simulink model "switching_mask"  (R2018a)
settings: Solver=FixedStepAuto  StartTime=0.0  StopTime=0.08  FixedStep=2.5000e-06  RelTol=1e-3
libraries: powerlib_meascontrol x11
settings Model: Creator=enes_  LastModifiedBy=enes_

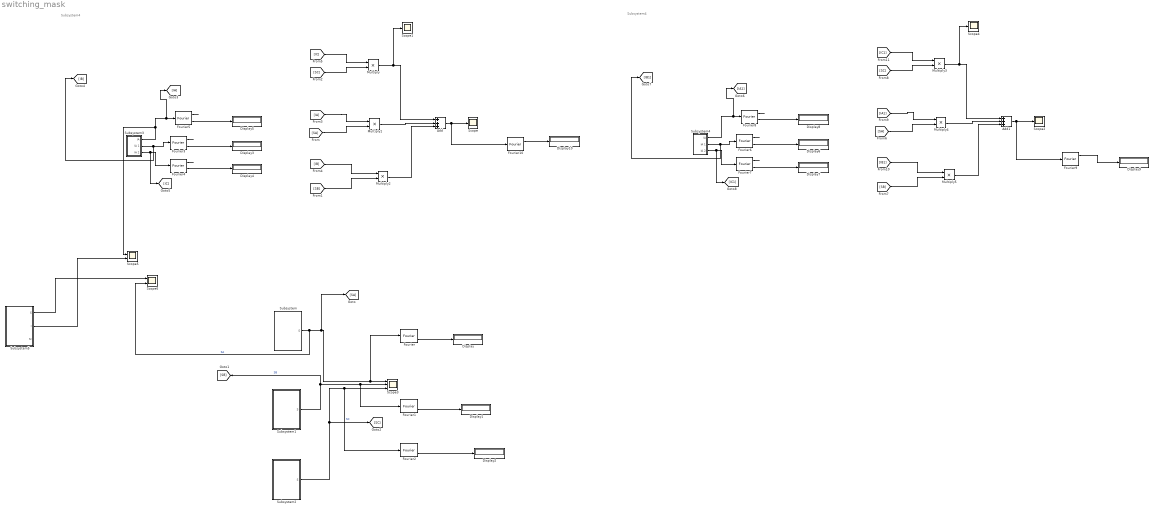
== system switching_mask ==
  note: Subsystem4
  note: Subsystem4
  Add : Sum  Inputs=3
  Add1 : Sum  Inputs=3
  Display{,1..10} (11 alike) : Display
  Fourier{,1..8} (9 alike) : powerlib_meascontrol/Measurements/Fourier  Freq=50  n=1  InInit=[0, 0]  Ts=0
      settings: SourceProductName=Simscape Power Systems
  Fourier10 : powerlib_meascontrol/Measurements/Fourier  Freq=100  n=1  InInit=[0, 0]  Ts=0
      settings: SourceProductName=Simscape Power Systems
  Fourier9 : powerlib_meascontrol/Measurements/Fourier  Freq=100  n=1  InInit=[0, 0]  Ts=0
      settings: SourceProductName=Simscape Power Systems
  Multiply{,1..5} (6 alike) : Product
  Scope{,1..2,4} (4 alike) : Scope
  Scope3 : Scope  NumInputPorts=3
  Scope5 : Scope  NumInputPorts=2
  Scope6 : Scope  NumInputPorts=2
  Subsystem : Subsystem  mask{m=0.9, f_s=4e4, f_f=50, the_f=0, the_c=0, i1=20, i2=5}
      mask prompts: m "modulation index"; f_s "carrier frequency"; f_f "fundemental frequency"; the_f "phase of fundamental"; the_c "phase of carrier"; i1 "iteration number of carrier"; i2 "iteration number of fundamental"
  Subsystem1 : Subsystem  mask{m=0.9, f_s=4e4, f_f=50, the_f=2*pi/3, the_c=0, i1=20, i2=5}
      mask prompts: m "modulation index"; f_s "carrier frequency"; f_f "fundemental frequency"; the_f "phase of fundamental"; the_c "phase of carrier"; i1 "iteration number of carrier"; i2 "iteration number of fundamental"
  Subsystem2 : Subsystem  mask{m=0.9, f_s=4e4, f_f=50, the_f=4*pi/3, the_c=0, i1=20, i2=5}
      mask prompts: m "modulation index"; f_s "carrier frequency"; f_f "fundemental frequency"; the_f "phase of fundamental"; the_c "phase of carrier"; i1 "iteration number of carrier"; i2 "iteration number of fundamental"
  Subsystem3 : Subsystem
  Subsystem4 : Subsystem
  Subsystem5 : Subsystem  mask{m=0.9, f_s=4e4, f_f=50, the_f=0, the_c=0, i1=20, i2=5, load_phase=pi/6}
      mask prompts: m "modulation index"; f_s "carrier frequency"; f_f "fundemental frequency"; the_f "phase of fundamental"; the_c "phase of carrier"; i1 "iteration number of carrier"; i2 "iteration number of fundamental"; load_phase "phase of load current"
  wires:
  Subsystem/1(S) -> Scope6/2, [SA], Fourier/1, Scope3/1  "SA"
  Subsystem1/1(S) -> [SB], Fourier1/1, Scope3/2  "SB"
  Subsystem2/1(S) -> [SC], Fourier2/1, Scope3/3  "SC"
  Fourier/2 -> Display/1
  Fourier1/2 -> Display1/1
  Fourier2/2 -> Display2/1
  Fourier3/1 -> ?
  [SC] -> Multiply/2
  [IA] -> Multiply1/1
  Subsystem3/1("IA ") -> Scope5/1, [IA], Fourier5/1
  Fourier5/2 -> Display5/1
  Multiply/1 -> Scope1/1, Add/1
  Fourier4/2 -> Display4/1
  Multiply1/1 -> Add/2
  [SB] -> Multiply2/2
  Fourier4/1 -> ?
  [SA] -> Multiply1/2
  [IB] -> Multiply2/1
  Subsystem3/2(IA 1) -> [IB], Fourier3/1
  Fourier5/1 -> ?
  Subsystem3/3(IA 2) -> [IC], Fourier4/1
  Multiply2/1 -> Add/3
  [IC] -> Multiply/1
  Fourier3/2 -> Display3/1
  Multiply3/1 -> Scope4/1, Add1/1
  [SC] -> Multiply3/2
  [IB1] -> Multiply5/1
  Fourier7/2 -> Display7/1
  Subsystem4/1("IA ") -> [IA1], Fourier8/1
  [IA1] -> Multiply4/1
  Fourier8/2 -> Display8/1
  Subsystem4/2(IA 1) -> [IB1], Fourier6/1
  Multiply5/1 -> Add1/3
  Subsystem4/3(IA 2) -> [IC1], Fourier7/1
  [SA] -> Multiply4/2
  Multiply4/1 -> Add1/2
  Fourier8/1 -> ?
  [SB] -> Multiply5/2
  Fourier6/1 -> ?
  Fourier6/2 -> Display6/1
  [IC1] -> Multiply3/1
  Fourier7/1 -> ?
  Add1/1 -> Fourier9/1, Scope2/1
  Fourier9/1 -> Display9/1
  Fourier10/1 -> Display10/1
  Add/1 -> Fourier10/1, Scope/1
  Subsystem5/2("I ") -> Scope5/2
  Subsystem5/1(S) -> Scope6/1

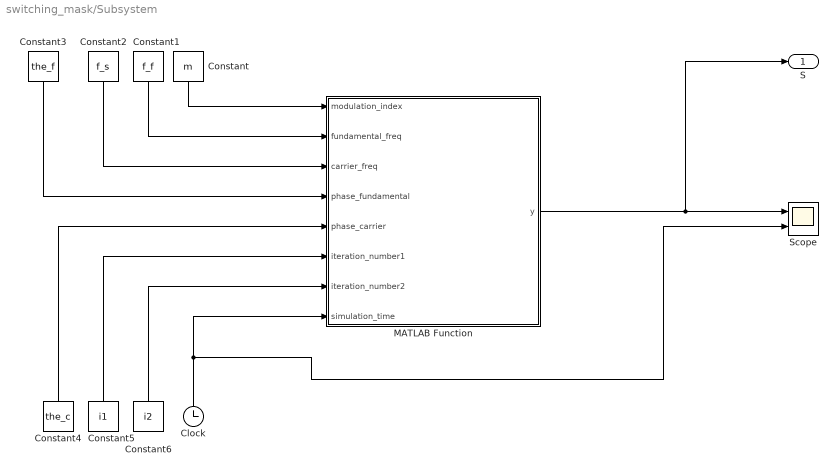
== system switching_mask/Subsystem ==
  Clock : Clock
  Constant : Constant  Value=m
  Constant1 : Constant  Value=f_f
  Constant2 : Constant  Value=f_s
  Constant3 : Constant  Value=the_f
  Constant4 : Constant  Value=the_c
  Constant5 : Constant  Value=i1
  Constant6 : Constant  Value=i2
  MATLAB Function : MATLAB Function  TreatAsAtomicUnit=on
  Scope : Scope  NumInputPorts=2
  S : Outport
  wires:
  Constant/1 -> MATLAB Function/1(modulation_index)
  Constant1/1 -> MATLAB Function/2(fundamental_freq)
  Constant2/1 -> MATLAB Function/3(carrier_freq)
  Constant3/1 -> MATLAB Function/4(phase_fundamental)
  Constant4/1 -> MATLAB Function/5(phase_carrier)
  Constant5/1 -> MATLAB Function/6(iteration_number1)
  Constant6/1 -> MATLAB Function/7(iteration_number2)
  MATLAB Function/1(y) -> S/1, Scope/1
  Clock/1 -> Scope/2, MATLAB Function/8(simulation_time)

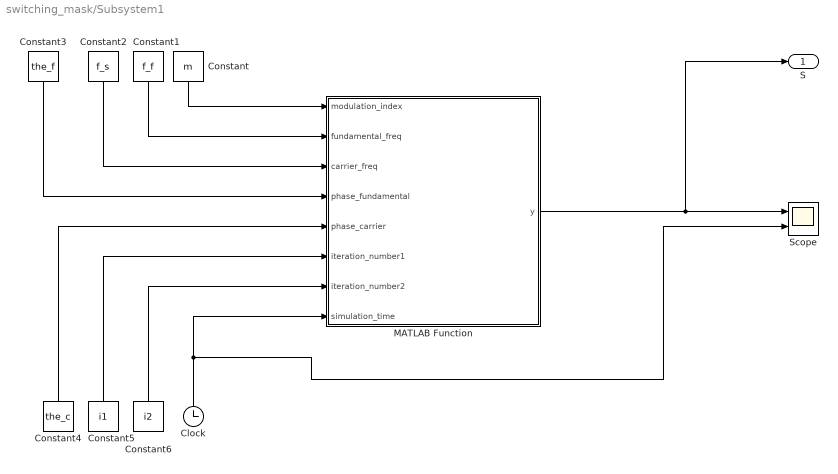
== system switching_mask/Subsystem1 ==
  Clock : Clock
  Constant : Constant  Value=m
  Constant1 : Constant  Value=f_f
  Constant2 : Constant  Value=f_s
  Constant3 : Constant  Value=the_f
  Constant4 : Constant  Value=the_c
  Constant5 : Constant  Value=i1
  Constant6 : Constant  Value=i2
  MATLAB Function : MATLAB Function  TreatAsAtomicUnit=on
  Scope : Scope  NumInputPorts=2
  S : Outport
  wires:
  Constant/1 -> MATLAB Function/1(modulation_index)
  Constant1/1 -> MATLAB Function/2(fundamental_freq)
  Constant2/1 -> MATLAB Function/3(carrier_freq)
  Constant3/1 -> MATLAB Function/4(phase_fundamental)
  Constant4/1 -> MATLAB Function/5(phase_carrier)
  Constant5/1 -> MATLAB Function/6(iteration_number1)
  Constant6/1 -> MATLAB Function/7(iteration_number2)
  MATLAB Function/1(y) -> S/1, Scope/1
  Clock/1 -> Scope/2, MATLAB Function/8(simulation_time)

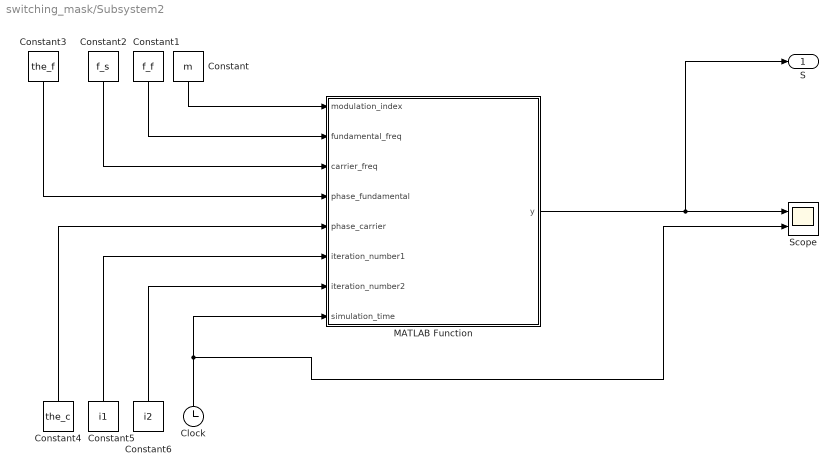
== system switching_mask/Subsystem2 ==
  Clock : Clock
  Constant : Constant  Value=m
  Constant1 : Constant  Value=f_f
  Constant2 : Constant  Value=f_s
  Constant3 : Constant  Value=the_f
  Constant4 : Constant  Value=the_c
  Constant5 : Constant  Value=i1
  Constant6 : Constant  Value=i2
  MATLAB Function : MATLAB Function  TreatAsAtomicUnit=on
  Scope : Scope  NumInputPorts=2
  S : Outport
  wires:
  Constant/1 -> MATLAB Function/1(modulation_index)
  Constant1/1 -> MATLAB Function/2(fundamental_freq)
  Constant2/1 -> MATLAB Function/3(carrier_freq)
  Constant3/1 -> MATLAB Function/4(phase_fundamental)
  Constant4/1 -> MATLAB Function/5(phase_carrier)
  Constant5/1 -> MATLAB Function/6(iteration_number1)
  Constant6/1 -> MATLAB Function/7(iteration_number2)
  MATLAB Function/1(y) -> S/1, Scope/1
  Clock/1 -> Scope/2, MATLAB Function/8(simulation_time)

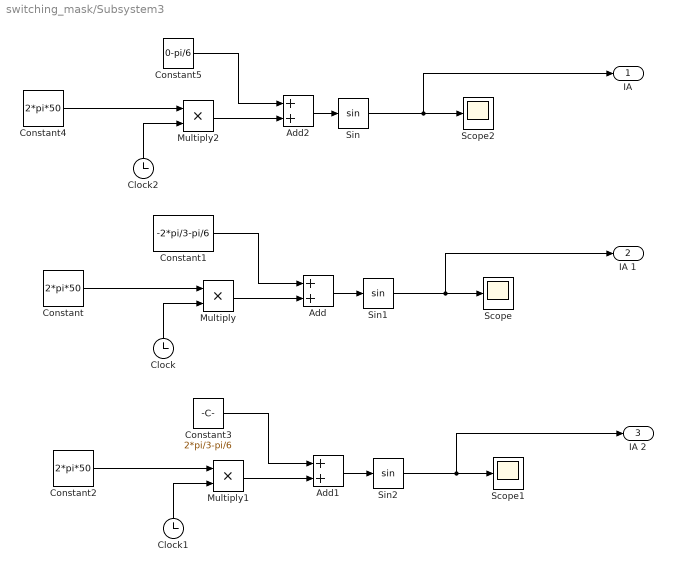
== system switching_mask/Subsystem3 ==
  Add : Sum
  Add1 : Sum
  Add2 : Sum
  Clock : Clock
  Clock1 : Clock
  Clock2 : Clock
  Constant : Constant  Value=2*pi*50
  Constant1 : Constant  Value=-2*pi/3-pi/6
  Constant2 : Constant  Value=2*pi*50
  Constant3 : Constant  Value=2*pi/3-pi/6
  Constant4 : Constant  Value=2*pi*50
  Constant5 : Constant  Value=0-pi/6
  Multiply : Product
  Multiply1 : Product
  Multiply2 : Product
  Scope : Scope
  Scope1 : Scope
  Scope2 : Scope
  Sin : Trigonometry
  Sin1 : Trigonometry
  Sin2 : Trigonometry
  "IA " : Outport
  IA 1 : Outport  Port=2
  IA 2 : Outport  Port=3
  wires:
  Multiply2/1 -> Add2/2
  Sin2/1 -> IA 2/1, Scope1/1
  Clock/1 -> Multiply/2
  Sin1/1 -> IA 1/1, Scope/1
  Sin/1 -> "IA "/1, Scope2/1
  Constant4/1 -> Multiply2/1
  Add/1 -> Sin1/1
  Constant3/1 -> Add1/1
  Clock2/1 -> Multiply2/2
  Add1/1 -> Sin2/1
  Constant2/1 -> Multiply1/1
  Clock1/1 -> Multiply1/2
  Multiply1/1 -> Add1/2
  Add2/1 -> Sin/1
  Constant1/1 -> Add/1
  Constant5/1 -> Add2/1
  Multiply/1 -> Add/2
  Constant/1 -> Multiply/1

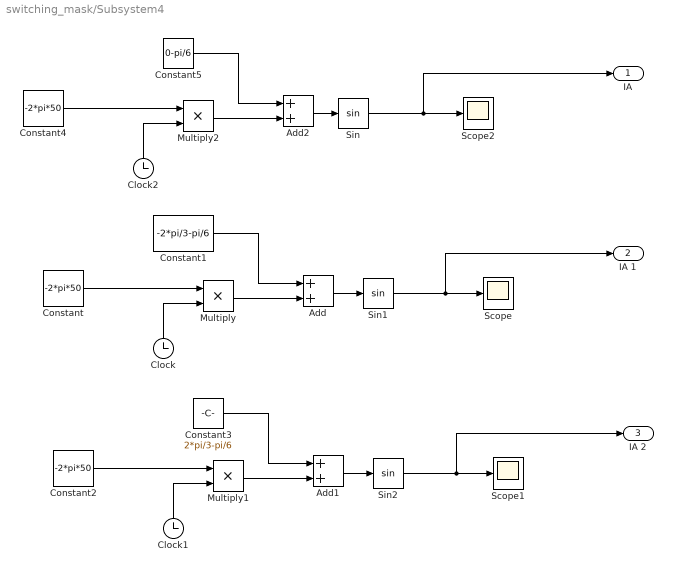
== system switching_mask/Subsystem4 ==
  Add : Sum
  Add1 : Sum
  Add2 : Sum
  Clock : Clock
  Clock1 : Clock
  Clock2 : Clock
  Constant : Constant  Value=-2*pi*50
  Constant1 : Constant  Value=-2*pi/3-pi/6
  Constant2 : Constant  Value=-2*pi*50
  Constant3 : Constant  Value=2*pi/3-pi/6
  Constant4 : Constant  Value=-2*pi*50
  Constant5 : Constant  Value=0-pi/6
  Multiply : Product
  Multiply1 : Product
  Multiply2 : Product
  Scope : Scope
  Scope1 : Scope
  Scope2 : Scope
  Sin : Trigonometry
  Sin1 : Trigonometry
  Sin2 : Trigonometry
  "IA " : Outport
  IA 1 : Outport  Port=2
  IA 2 : Outport  Port=3
  wires:
  Multiply2/1 -> Add2/2
  Sin2/1 -> IA 2/1, Scope1/1
  Clock/1 -> Multiply/2
  Sin1/1 -> IA 1/1, Scope/1
  Sin/1 -> "IA "/1, Scope2/1
  Constant4/1 -> Multiply2/1
  Add/1 -> Sin1/1
  Constant3/1 -> Add1/1
  Clock2/1 -> Multiply2/2
  Add1/1 -> Sin2/1
  Constant2/1 -> Multiply1/1
  Clock1/1 -> Multiply1/2
  Multiply1/1 -> Add1/2
  Add2/1 -> Sin/1
  Constant1/1 -> Add/1
  Constant5/1 -> Add2/1
  Multiply/1 -> Add/2
  Constant/1 -> Multiply/1

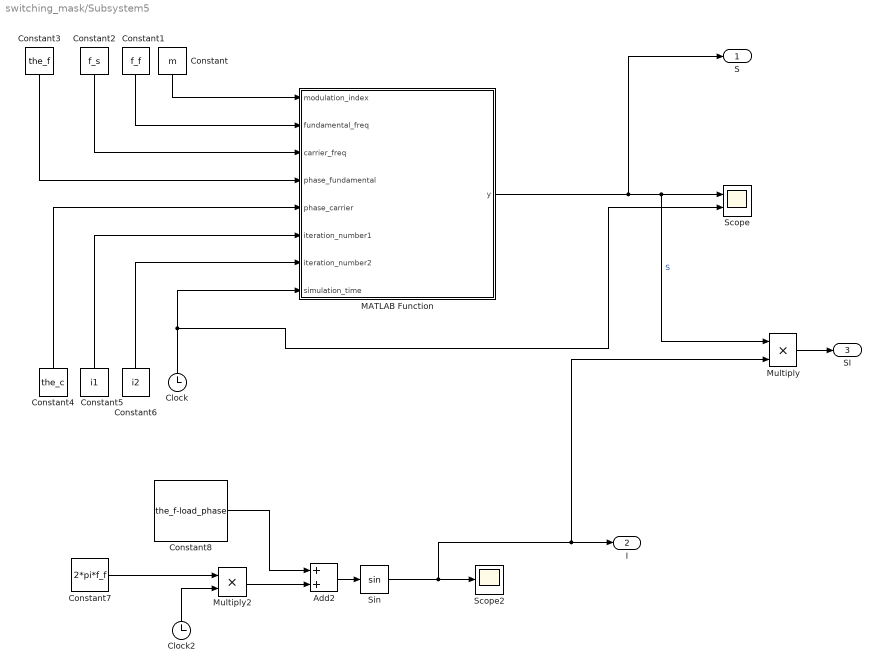
== system switching_mask/Subsystem5 ==
  Add2 : Sum
  Clock : Clock
  Clock2 : Clock
  Constant : Constant  Value=m
  Constant1 : Constant  Value=f_f
  Constant2 : Constant  Value=f_s
  Constant3 : Constant  Value=the_f
  Constant4 : Constant  Value=the_c
  Constant5 : Constant  Value=i1
  Constant6 : Constant  Value=i2
  Constant7 : Constant  Value=2*pi*f_f
  Constant8 : Constant  Value=the_f-load_phase
  MATLAB Function : MATLAB Function  TreatAsAtomicUnit=on
  Multiply : Product
  Multiply2 : Product
  Scope : Scope  NumInputPorts=2
  Scope2 : Scope
  Sin : Trigonometry
  S : Outport
  "I " : Outport  Port=2
  SI : Outport  Port=3
  wires:
  Constant/1 -> MATLAB Function/1(modulation_index)
  Constant1/1 -> MATLAB Function/2(fundamental_freq)
  Constant2/1 -> MATLAB Function/3(carrier_freq)
  Constant3/1 -> MATLAB Function/4(phase_fundamental)
  Constant4/1 -> MATLAB Function/5(phase_carrier)
  Constant5/1 -> MATLAB Function/6(iteration_number1)
  Constant6/1 -> MATLAB Function/7(iteration_number2)
  MATLAB Function/1(y) -> S/1, Multiply/1, Scope/1  "S"
  Clock/1 -> Scope/2, MATLAB Function/8(simulation_time)
  Constant7/1 -> Multiply2/1
  Sin/1 -> Multiply/2, "I "/1, Scope2/1
  Add2/1 -> Sin/1
  Clock2/1 -> Multiply2/2
  Constant8/1 -> Add2/1
  Multiply2/1 -> Add2/2
  Multiply/1 -> SI/1

== matlab function switching_mask/Subsystem1/MATLAB Function ==
  data: modulation_index input; y output; fundamental_freq input; carrier_freq input; phase_fundamental input; phase_carrier input; iteration_number1 input; iteration_number2 input; simulation_time input
function y  = fcn(modulation_index, fundamental_freq,carrier_freq,phase_fundamental, phase_carrier, iteration_number1,iteration_number2,simulation_time)

y=0;

fundamental_angFreq=2*pi*fundamental_freq;
carrier_angFreq= 2*pi*carrier_freq;
phase_fundamental=phase_fundamental+pi/2;


for m=1:iteration_number1
    for n= -iteration_number2:iteration_number2  
        k=(2/(m*pi))*sin((m+n)*pi/2)*...
                besselj(n,m*modulation_index*pi/2)*...
                cos(m*(carrier_angFreq*simulation_time-phase_carrier)...
                +n*(fundamental_angFreq*simulation_time-phase_fundamental));
       y=y+real(k);
          
        
        
    end
end

y= y+(1/2)+ (modulation_index/2)*cos(fundamental_angFreq*simulation_time-phase_fundamental);

== matlab function switching_mask/Subsystem/MATLAB Function ==
  data: modulation_index input; y output; fundamental_freq input; carrier_freq input; phase_fundamental input; phase_carrier input; iteration_number1 input; iteration_number2 input; simulation_time input
function y  = fcn(modulation_index, fundamental_freq,carrier_freq,phase_fundamental, phase_carrier, iteration_number1,iteration_number2,simulation_time)

y=0;

fundamental_angFreq=2*pi*fundamental_freq;
carrier_angFreq= 2*pi*carrier_freq;
phase_fundamental=phase_fundamental+pi/2;


for m=1:iteration_number1
    for n= -iteration_number2:iteration_number2  
        k=(2/(m*pi))*sin((m+n)*pi/2)*...
                besselj(n,m*modulation_index*pi/2)*...
                cos(m*(carrier_angFreq*simulation_time-phase_carrier)...
                +n*(fundamental_angFreq*simulation_time-phase_fundamental));
       y=y+real(k);
          
        
        
    end
end

y= y+(1/2)+ (modulation_index/2)*cos(fundamental_angFreq*simulation_time-phase_fundamental);

== matlab function switching_mask/Subsystem2/MATLAB Function ==
  data: modulation_index input; y output; fundamental_freq input; carrier_freq input; phase_fundamental input; phase_carrier input; iteration_number1 input; iteration_number2 input; simulation_time input
function y  = fcn(modulation_index, fundamental_freq,carrier_freq,phase_fundamental, phase_carrier, iteration_number1,iteration_number2,simulation_time)

y=0;

fundamental_angFreq=2*pi*fundamental_freq;
carrier_angFreq= 2*pi*carrier_freq;
phase_fundamental=phase_fundamental+pi/2;


for m=1:iteration_number1
    for n= -iteration_number2:iteration_number2  
        k=(2/(m*pi))*sin((m+n)*pi/2)*...
                besselj(n,m*modulation_index*pi/2)*...
                cos(m*(carrier_angFreq*simulation_time-phase_carrier)...
                +n*(fundamental_angFreq*simulation_time-phase_fundamental));
       y=y+real(k);
          
        
        
    end
end

y= y+(1/2)+ (modulation_index/2)*cos(fundamental_angFreq*simulation_time-phase_fundamental);

== matlab function switching_mask/Subsystem5/MATLAB Function ==
  data: modulation_index input; y output; fundamental_freq input; carrier_freq input; phase_fundamental input; phase_carrier input; iteration_number1 input; iteration_number2 input; simulation_time input
function y  = fcn(modulation_index, fundamental_freq,carrier_freq,phase_fundamental, phase_carrier, iteration_number1,iteration_number2,simulation_time)

y=0;

fundamental_angFreq=2*pi*fundamental_freq;
carrier_angFreq= 2*pi*carrier_freq;
phase_fundamental=phase_fundamental+pi/2;


for m=1:iteration_number1
    for n= -iteration_number2:iteration_number2  
        k=(2/(m*pi))*sin((m+n)*pi/2)*...
                besselj(n,m*modulation_index*pi/2)*...
                cos(m*(carrier_angFreq*simulation_time-phase_carrier)...
                +n*(fundamental_angFreq*simulation_time-phase_fundamental));
       y=y+real(k);
          
        
        
    end
end

y= y+(1/2)+ (modulation_index/2)*cos(fundamental_angFreq*simulation_time-phase_fundamental);
